simulink model "experimentalTensorCommDeserializeMultiTensor"  (R2023b)
settings: Solver=VariableStepAuto  StartTime=0.0  StopTime=10.0  RelTol=1e-3
libraries: instrumentlib x2
settings Model: Creator=peterc  LastModifiedBy=peterc

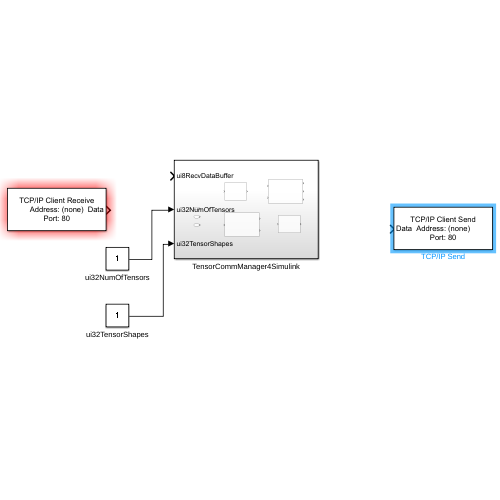
[thumbnail: Simulink's stored preview of the top-level diagram]
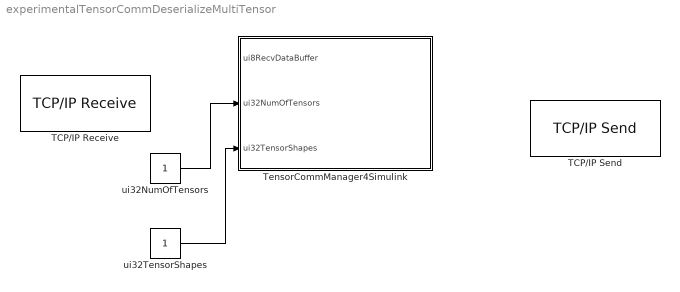
== system experimentalTensorCommDeserializeMultiTensor ==
  TCP/IP Receive : instrumentlib/TCP//IP Receive  Port=80  DataSize=dTotalBufferSize  DataType=uint8  ASCIIFormatting=%f  Terminator=LF  CustomTerminator=10  ByteOrder=big-endian  EnableBlockingMode=on  Timeout=60  SampleTime=0.01  SimulateUsing=Interpreted execution
  TCP/IP Send : instrumentlib/TCP//IP Send  Port=80  ByteOrder=little-endian  EnableBlockingMode=on  Timeout=10  TransferDelay=off  SimulateUsing=Interpreted execution
  TensorCommManager4Simulink : Subsystem
  ui32NumOfTensors : Constant
  ui32TensorShapes : Constant
  wires:
  ui32NumOfTensors/1 -> TensorCommManager4Simulink/2(ui32NumOfTensors)
  ui32TensorShapes/1 -> TensorCommManager4Simulink/3(ui32TensorShapes)

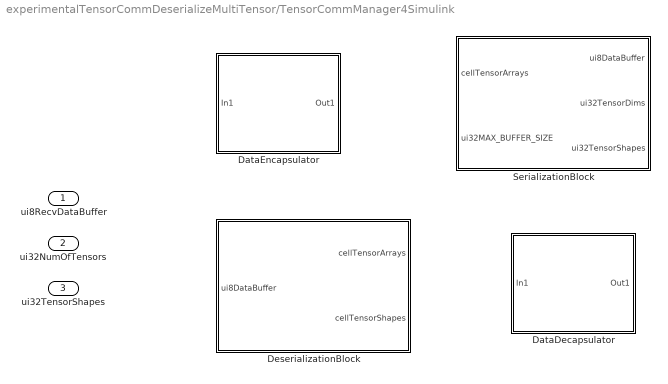
== system experimentalTensorCommDeserializeMultiTensor/TensorCommManager4Simulink ==
  ui8RecvDataBuffer : Inport
  ui32NumOfTensors : Inport  Port=2
  ui32TensorShapes : Inport  Port=3
  DataDecapsulator : Subsystem
  DataEncapsulator : Subsystem
  DeserializationBlock : MATLAB Function  TreatAsAtomicUnit=on
  SerializationBlock : MATLAB Function  TreatAsAtomicUnit=on

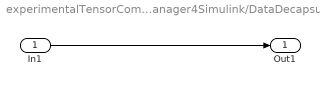
== system experimentalTensorCommDeserializeMultiTensor/TensorCommManager4Simulink/DataDecapsulator ==
  In1 : Inport
  Out1 : Outport
  wires:
  In1/1 -> Out1/1

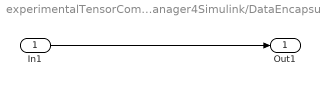
== system experimentalTensorCommDeserializeMultiTensor/TensorCommManager4Simulink/DataEncapsulator ==
  In1 : Inport
  Out1 : Outport
  wires:
  In1/1 -> Out1/1

== matlab function experimentalTensorCommDeserializeMultiTensor/TensorCommManager4Simulink/SerializationBlock ==
  data: cellTensorArrays input; ui8DataBuffer output; ui32TensorDims output; ui32MAX_BUFFER_SIZE input; ui32TensorShapes output
function [ui8DataBuffer, ui32TensorDims, ui32TensorShapes] = MultiTensor2Bytes(cellTensorArrays, ui32MAX_BUFFER_SIZE)
arguments
    cellTensorArrays {mustBeA(cellTensorArrays, ["cell","double","uint8","single"])}
    ui32MAX_BUFFER_SIZE (1,1) uint32 {isnumeric, isscalar} = 1E8
end
%% SIGNATURE
% [ui8DataBuffer, ui32TensorDims, ui32TensorShapes] = MultiTensor2Bytes(cellTensorArrays, kwargs)
% -------------------------------------------------------------------------------------------------------------
%% DESCRIPTION
% What the function does
% -------------------------------------------------------------------------------------------------------------
%% INPUT
% in1 [dim] description
% Name1                     []
% Name2                     []
% Name3                     []
% -------------------------------------------------------------------------------------------------------------
%% OUTPUT
% out1 [dim] description
% Name1                     []
% Name2                     []
% Name3                     []
% -------------------------------------------------------------------------------------------------------------
%% CHANGELOG
% 18-12-2024        Pietro Califano       First implementation (ported from python)
% -------------------------------------------------------------------------------------------------------------

% Input detected to be a tensor, perform wrapping to cell
if isnumeric(cellTensorArrays)
    cellTensorArrays = {cellTensorArrays};
end

% Get number of tensors in cell
ui32NumOfTensors = uint32(length(cellTensorArrays));

ui8DataBuffer = zeros(1, ui32MAX_BUFFER_SIZE, 'uint8');
ui64BufferAllocPtr = uint64(1);

ui32TensorDims   = cell(1, ui32NumOfTensors);
ui32TensorShapes = cell(1, ui32NumOfTensors);

ui64TmpMsgEndPtr = uint64(0);

% Build multi-tensor message
for idMsg = 1:ui32NumOfTensors

    tmpMsgBuffer = TensorArray2Bytes( cellTensorArrays{idMsg} );
    ui64TmpMsgEndPtr = ui64TmpMsgEndPtr + uint64(length(tmpMsgBuffer));

    % Allocate message
    ui8DataBuffer(ui64BufferAllocPtr : ui64TmpMsgEndPtr) =  tmpMsgBuffer;

    % Update allocation ptr
    ui64BufferAllocPtr = ui64TmpMsgEndPtr + 1;
end

% Remove unused bytes
ui8DataBuffer = ui8DataBuffer(1:ui64BufferAllocPtr-1);

% Add number of tensors to message header
ui8DataBuffer = [typecast(ui32NumOfTensors, 'uint8'), ui8DataBuffer];

%% LOCAL FUNCTION
    function [ui8DataBuffer, ui32TensorDims, ui32TensorShape] = TensorArray2Bytes(dTensorArray, ui32NumOfBatches, ui32NumOfChannels)
        % arguments
        %     dTensorArray double
        % end
        % arguments
        %     kwargs.ui32NumOfBatches  (1,1) uint32 {isscalar} = 0
        %     kwargs.ui32NumOfChannels (1,1) uint32 {isscalar} = 0
        % end

        %% FUNCTIONS
        % COPY FROM HERE
        %% SIGNATURE
        % -------------------------------------------------------------------------------------------------------------
        %% DESCRIPTION
        % What the function does
        % -------------------------------------------------------------------------------------------------------------
        %% INPUT
        % in1 [dim] description
        % Name1                     []
        % Name2                     []
        % Name3                     []
        % -------------------------------------------------------------------------------------------------------------
        %% OUTPUT
        % out1 [dim] description
        % Name1                     []
        % Name2                     []
        % Name3                     []
        % -------------------------------------------------------------------------------------------------------------
        %% CHANGELOG
        % 01-12-2024        Pietro Califano       First implementation (ported from python)
        % 17-12-2024        Pietro Califano       Validation and unit testing completed
        % -------------------------------------------------------------------------------------------------------------

        % Static method to convert tensor array (N-dim array) to buffer of bytes to transmit over TCP (format tailored for PyTorchAutoForge)

        % Get tensor shape
        ui32TensorShape = uint32(size(dTensorArray));

        % Get number of dimensions
        ui32TensorDims = uint32(length(ui32TensorShape));

        % If specified, add number of batches and channels to shape
        if ui32NumOfBatches > 0
            ui32TensorShape = [ui32NumOfBatches, ui32TensorShape];
            ui32TensorDims = ui32TensorDims + 1;
        end

        if ui32NumOfChannels > 0
            ui32TensorShape = [ui32TensorShape, ui32NumOfChannels];
            ui32TensorDims = ui32TensorDims + 1;
        end

        % Flatten tensor data to linear array and downcast to single
        fTensorBuffer = single(dTensorArray(:));

        % Convert tensor data to bytes
        ui8TensorBuffer = typecast(fTensorBuffer, 'uint8');

        if iscolumn(ui8TensorBuffer)
            ui8TensorBuffer = ui8TensorBuffer';
        end

        % Convert tensor shape to bytes
        ui8TensorDims = typecast(ui32TensorDims, 'uint8');
        ui8TensorShape = typecast(ui32TensorShape, 'uint8');

        % Construct data buffer
        ui8DataBuffer = [ui8TensorDims, ui8TensorShape, ui8TensorBuffer];

        % Add message length to buffer
        ui32MessageBytes = uint32(length(ui8DataBuffer));
        ui8DataBuffer = [typecast(ui32MessageBytes, 'uint8'), ui8DataBuffer];

    end
end

== matlab function experimentalTensorCommDeserializeMultiTensor/TensorCommManager4Simulink/DeserializationBlock ==
  data: ui8DataBuffer input; cellTensorArrays output; cellTensorShapes output
function [cellTensorArrays, cellTensorShapes] = Bytes2MultiTensor(ui8DataBuffer)
arguments
    ui8DataBuffer        (1,:) uint8 {isscalar, isa(ui8DataBuffer, 'uint8')}
end
%% SIGNATURE
% -------------------------------------------------------------------------------------------------------------
%% DESCRIPTION
% What the function does
% -------------------------------------------------------------------------------------------------------------
%% INPUT
% in1 [dim] description
% Name1                     []
% Name2                     []
% Name3                     []
% -------------------------------------------------------------------------------------------------------------
%% OUTPUT
% out1 [dim] description
% Name1                     []
% Name2                     []
% Name3                     []
% -------------------------------------------------------------------------------------------------------------
%% CHANGELOG
% 18-12-2024        Pietro Califano       First implementation (ported from python)
% -------------------------------------------------------------------------------------------------------------

% numOfTensors = int.from_bytes(inputDataBuffer[:4], self.ENDIANNESS)

% Get number of tensors to unpack
ui32NumOfTensors = typecast(ui8DataBuffer(1:4), 'uint32');

% Define output cell
cellTensorArrays = cell(1, ui32NumOfTensors);
cellTensorShapes = cell(1, ui32NumOfTensors);

ui64UnpackPtr = uint64(5);

% Unpack each message separately
for idMsg = 1:ui32NumOfTensors

    % # Get length of tensor message
    % tensorMessageLength = int.from_bytes(inputDataBuffer[ptrStart:ptrStart+4], self.ENDIANNESS) # In bytes
    ui32TensorMessageLength = typecast(ui8DataBuffer(ui64UnpackPtr:ui64UnpackPtr+3), 'uint32');

    fprintf("\nProcessing Tensor message of length: %d\n", ui32TensorMessageLength)

    % # Extract sub-message from buffer
    % subTensorMessage = inputDataBuffer[ptrStart+4:(ptrStart + 4) + tensorMessageLength] # Extract sub-message in bytes
    ui8SubTensorMessage = ui8DataBuffer(ui64UnpackPtr + 4 : ui64UnpackPtr + 3 + uint64(ui32TensorMessageLength));

    % # Call function to convert each tensor message to tensor
    % tensor, tensorShape = self.BytesBufferToTensor(subTensorMessage)
    [dTensorArray, ~, i32TensorShape] = Bytes2TensorArray(ui32TensorMessageLength, ui8SubTensorMessage);

    % Append to cell
    cellTensorArrays{idMsg} = dTensorArray;
    cellTensorShapes{idMsg} = i32TensorShape;

    % Update buffer ptr for next tensor message
    % ptrStart = (ptrStart + 4) + tensorMessageLength
    ui64UnpackPtr = ui64UnpackPtr + uint64(4) + uint64(ui32TensorMessageLength);
end

%% LOCAL FUNCTION
    function [dTensorArray, i32TensorDims, i32TensorShape] = Bytes2TensorArray(ui32RecvMessageBytes, ui8DataBuffer)
        % arguments
        %     ui32RecvMessageBytes (1, 1) uint32 {isscalar}
        %     ui8DataBuffer (1, :) uint8  {isvector}
        % end
        %% FUNCTIONS
        % COPY FROM HERE
        %% SIGNATURE
        % -------------------------------------------------------------------------------------------------------------
        %% DESCRIPTION
        % What the function does
        % -------------------------------------------------------------------------------------------------------------
        %% INPUT
        % in1 [dim] description
        % Name1                     []
        % Name2                     []
        % Name3                     []
        % -------------------------------------------------------------------------------------------------------------
        %% OUTPUT
        % out1 [dim] description
        % Name1                     []
        % Name2                     []
        % Name3                     []
        % -------------------------------------------------------------------------------------------------------------
        %% CHANGELOG
        % 01-12-2024        Pietro Califano       First implementation (ported from python)
        % 17-12-2024        Pietro Califano       Validation and unit testing completed
        % -------------------------------------------------------------------------------------------------------------

        % Static method to convert buffer of bytes to tensor array (N-dim array) (format tailored for PyTorchAutoForge)

        % Read bytes indicating how many sizes are to unpack
        i32TensorDims = typecast(ui8DataBuffer(1:4), 'uint32');

        % Create shape array
        i32TensorShape = zeros(1, i32TensorDims, "uint32");

        for idPtr = 1:i32TensorDims
            i32TensorShape(idPtr) = typecast(ui8DataBuffer(4*idPtr+1:4*idPtr+4), 'uint32');
        end

        % Assign idPtr to next byte
        idPtr = 4*i32TensorDims + 4; % TBC

        % Check ptr is lower than total bytes
        assert(idPtr < ui32RecvMessageBytes, 'ERROR: Pointer exceeds total bytes.')

        % Get bytes of tensor data from buffer and do typecasting
        dTensorBuffer = typecast(ui8DataBuffer(idPtr+1:end), 'single');

        assert(length(dTensorBuffer) <= length(ui8DataBuffer(idPtr+1:end)), 'ACHTUNG: message typecast failed!');

        % Reshape tensor data according to i32TensorShape
        dTensorArray = reshape(dTensorBuffer, i32TensorShape);

        % Squeeze tensor if any dimension is 1
        if any(i32TensorShape == 1)
            dTensorArray = squeeze(dTensorArray);
        end

    end


end
